simulink model "lqrproyecto1"  (R2018a)
settings: Solver=VariableStepAuto  StartTime=0.0  StopTime=10.0  RelTol=1e-3
settings Model: Creator=Alvaro  LastModifiedBy=Alvaro

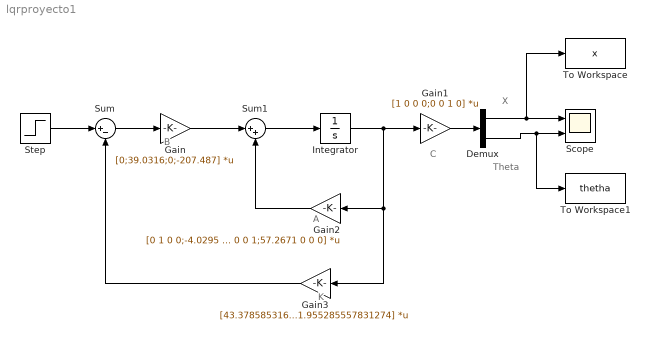
== system lqrproyecto1 ==
  note: X
  note: Theta
  note: K
  note: C
  note: A
  note: B
  Demux : Demux  Outputs=2
  Gain : Gain  Gain=[0;39.0316;0;-207.487]  Multiplication=Matrix(K*u)
  Gain1 : Gain  Gain=[1 0 0 0;0 0 1 0]  Multiplication=Matrix(K*u)
  Gain2 : Gain  Gain=[0 1 0 0;-4.0295 0 0 0;0 0 0 1;57.2671 0 0 0]  Multiplication=Matrix(K*u)
  Gain3 : Gain  Gain=[43.37858531679103 16.9900283404516 1.060660171797636 1.955285557831274]  Multiplication=Matrix(K*u)
  Integrator : Integrator  InitialCondition=[0,0.1,0,0.1]
  Scope : Scope  NumInputPorts=2
  Step : Step  Time=0  After=0  SampleTime=0
  Sum : Sum  Inputs=|+-
  Sum1 : Sum  Inputs=|++
  To Workspace : ToWorkspace  VariableName=x  SampleTime=-1
  To Workspace1 : ToWorkspace  VariableName=thetha  SampleTime=-1
  wires:
  Sum/1 -> Gain/1
  Gain/1 -> Sum1/1
  Sum1/1 -> Integrator/1
  Integrator/1 -> Gain3/1, Gain2/1, Gain1/1
  Gain1/1 -> Demux/1
  Gain2/1 -> Sum1/2
  Gain3/1 -> Sum/2
  Step/1 -> Sum/1
  Demux/1 -> To Workspace/1, Scope/1
  Demux/2 -> To Workspace1/1, Scope/2
